simulink model "IPC4M"  (R2015a)
settings: Solver=ode3  SolverMode=SingleTasking  StartTime=0.0  StopTime=10.0  FixedStep=1e-2  RelTol=1e-7
values from neighbouring files (symbols this model uses):
  d1 = 70    [IPC4Minit.m]
  d2 = 70    [IPC4Minit.m]
  d3 = 70    [IPC4Minit.m]
  d4 = 70    [IPC4Minit.m]
  delta1 = 9    [IPC4Minit.m]
  delta2 = 9    [IPC4Minit.m]
  delta3 = 9    [IPC4Minit.m]
  delta4 = 9    [IPC4Minit.m]
  g = [0;0;-9.81]    [IPC4Minit.m]
  j0 = 10    [IPC4Minit.m]
  j1 = 10    [IPC4Minit.m]
  j1d = 1.00*j1    (= 10)    [IPC4Minit.m]
  j2 = 10    [IPC4Minit.m]
  j2d = 1.00*j2    (= 10)    [IPC4Minit.m]
  j3 = 10    [IPC4Minit.m]
  j3d = 1.00*j3    (= 10)    [IPC4Minit.m]
  j4 = 10    [IPC4Minit.m]
  j4d = 1.00*j4    (= 10)    [IPC4Minit.m]
  k1 = 2000    [IPC4Minit.m]
  k2 = 2000    [IPC4Minit.m]
  k3 = 2000    [IPC4Minit.m]
  k4 = 2000    [IPC4Minit.m]
  kappa1 = 10    [IPC4Minit.m]
  kappa2 = 10    [IPC4Minit.m]
  kappa3 = 10    [IPC4Minit.m]
  kappa4 = 10    [IPC4Minit.m]
  Kc = 150    [IPC4Minit.m]
  l = [1 1 1 1]    [IPC4Minit.m]
  m0 = 10    [IPC4Minit.m]
  m1 = 10    [IPC4Minit.m]
  m1d = 0.00*m1    (= 0)    [IPC4Minit.m]
  m2 = 10    [IPC4Minit.m]
  m2d = 0.00*m2    (= 0)    [IPC4Minit.m]
  m3 = 10    [IPC4Minit.m]
  m3d = 0.00*m3    (= 0)    [IPC4Minit.m]
  m4 = 10    [IPC4Minit.m]
  m4d = 0.00*m4    (= 0)    [IPC4Minit.m]
libraries: aerolibutil x11, dspinverses x3
(part 1 of 3)
settings Model: CovSFcnEnable=off  Creator=Martin  LastModifiedBy=mangerer
settings SolverCC: ZeroCrossAlgorithm=Adaptive
settings DataIOCC: LimitDataPoints=off
settings OptimizationCC: BlockReduction=off  BooleanDataType=off
settings DebuggingCC: SaveWithParameterizedLinksMsg=none  UnderspecifiedInitializationDetection=Classic  MergeDetectMultiDrivingBlocksExec=none  SignalResolutionControl=TryResolveAllWithWarning
settings HardwareCC: TargetUnknown=on

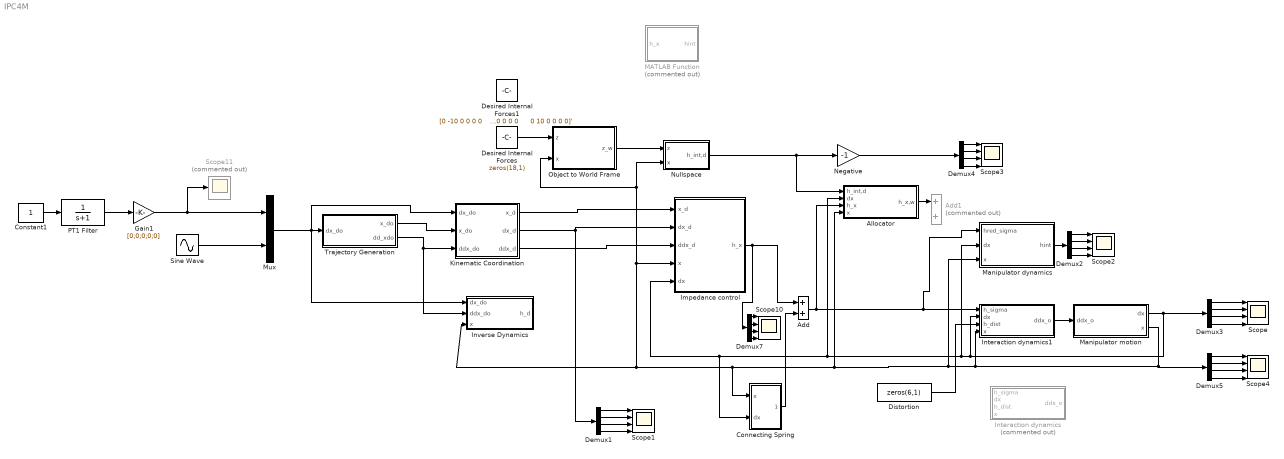
== system IPC4M ==
  Add : Sum
  Add1 : Sum  Commented=on
  Allocator : Subsystem
  Connecting Spring : Subsystem
  Constant1 : Constant
  Demux{1..5,7} (6 alike) : Demux
  Desired Internal Forces : Constant  Value=zeros(18,1)
  Desired Internal Forces1 : Constant  Value="[0 -10 0 0 0 0    10 0 0 0 0 0      0 10 0 0 0 0]'"
  Distortion : Constant  Value=zeros(6,1)
  Gain1 : Gain  Gain=[0;0;0;0;0]
  Impedance control : Subsystem
  Interaction dynamics : Subsystem  Commented=on
  Interaction dynamics1 : Subsystem
  Inverse Dynamics : Subsystem
  Kinematic Coordination : Subsystem
  MATLAB Function : MATLAB Function  Commented=on  TreatAsAtomicUnit=on
  Manipulator dynamics : Subsystem
  Manipulator motion : Subsystem
  Mux : Mux  Inputs=2
  Negative : Gain  Gain=-1
  Nullspace : Subsystem
  Object to World Frame : MATLAB Function  TreatAsAtomicUnit=on
  PT1 Filter : TransferFcn  Denominator=[1 1]
  Scope{,1..4,10} (6 alike) : Scope  NumInputPorts=4
      Scope settings: ShowLegends=on  YMin=-0.25~-0.25~-0.25~-0.25  YMax=2~2~2~2
      Scope1 settings: ShowLegends=on  YMin=-1.5~-1.5~-1.5~-1.5  YMax=6~5.5~6~5.5
      Scope10 settings: ShowLegends=on  YMin=-75~-75~-75~-75  YMax=75~75~75~75  SaveName=ScopeData18
      Scope2 settings: ShowLegends=on  YMin=-150~-150~-150~-150  YMax=150~150~150~150  SaveName=ScopeData2
      Scope3 settings: ShowLegends=on  YMin=-5~-5~-5~-5  YMax=5~5~5~5  SaveName=ScopeData8
      Scope4 settings: ShowLegends=on  YMin=-5~-5~-5~-5  YMax=5~5~5~5  SaveName=ScopeData10
  Scope11 : Scope  Commented=on
      settings: YMin=0.9984  YMax=1  SaveName=ScopeData26
  Sine Wave : Sin  Frequency=1*pi  SampleTime=0
  Trajectory Generation : Subsystem
  wires:
  Manipulator dynamics/1(hint) -> Demux2/1
  Demux2/1 -> Scope2/1
  Demux2/2 -> Scope2/2
  Demux2/4 -> Scope2/4
  Demux3/1 -> Scope/1
  Demux3/2 -> Scope/2
  Demux3/3 -> Scope/3
  Demux3/4 -> Scope/4
  Demux5/1 -> Scope4/1
  Demux5/2 -> Scope4/2
  Demux5/3 -> Scope4/3
  Demux5/4 -> Scope4/4
  Object to World Frame/1(z_w) -> Nullspace/1(z)
  Nullspace/1(h_int,d) -> Negative/1, Allocator/1(h_int,d)
  Demux7/1 -> Scope10/1
  Demux7/2 -> Scope10/2
  Demux7/3 -> Scope10/3
  Demux7/4 -> Scope10/4
  PT1 Filter/1 -> Gain1/1
  Gain1/1 -> Mux/1, Scope11/1
  Impedance control/1(h_x) -> Demux7/1, Add/1
  Manipulator motion/1(dx) -> Demux3/1, Connecting Spring/2(dx), Impedance control/5(dx), Allocator/2(dx), Manipulator dynamics/2(dx), Interaction dynamics1/2(dx)
  Trajectory Generation/2(dd_xdo) -> Inverse Dynamics/2(ddx_do), Kinematic Coordination/3(ddx_do)
  Trajectory Generation/1(x_do) -> Kinematic Coordination/2(x_do)
  Mux/1 -> Inverse Dynamics/1(dx_do), Kinematic Coordination/1(dx_do), Trajectory Generation/1(dx_do)
  Kinematic Coordination/1(x_d) -> Impedance control/1(x_d)
  Kinematic Coordination/3(ddx_d) -> Impedance control/3(ddx_d)
  Manipulator motion/2(x) -> Demux5/1, Connecting Spring/1(x), Inverse Dynamics/3(x), Object to World Frame/2(x), Nullspace/2(x), Impedance control/4(x), Allocator/4(x), Manipulator dynamics/3(x), Interaction dynamics1/4(x)
  Constant1/1 -> PT1 Filter/1
  Demux1/1 -> Scope1/1
  Demux1/2 -> Scope1/2
  Demux1/3 -> Scope1/3
  Demux1/4 -> Scope1/4
  Kinematic Coordination/2(dx_d) -> Impedance control/2(dx_d), Demux1/1
  Negative/1 -> Demux4/1
  Demux4/1 -> Scope3/1
  Demux4/2 -> Scope3/2
  Demux4/4 -> Scope3/4
  Sine Wave/1 -> Mux/2
  Demux2/3 -> Scope2/3
  Demux4/3 -> Scope3/3
  Desired Internal Forces/1 -> Object to World Frame/1(z)
  Add/1 -> Allocator/3(h_x), Manipulator dynamics/1(hred_sigma), Interaction dynamics1/1(h_sigma)
  Interaction dynamics1/1(ddx_o) -> Manipulator motion/1(ddx_o)
  Distortion/1 -> Interaction dynamics1/3(h_dist)
  Connecting Spring/1(h_con) -> Add/2
  Allocator/1(h_x,w) -> Add1/1

== system IPC4M/Allocator ==
  h_int,d : Inport
  dx : Inport  Port=2
  h_x : Inport  Port=3
  x : Inport  Port=4
  Add : Sum  Inputs=-+
  Add1 : Sum
  Divide : Product  Inputs=*/*  Multiplication=Matrix(*)
  Divide1 : Product  Inputs=*/*  Multiplication=Matrix(*)
  Divide2 : Product  Inputs=*/*  Multiplication=Matrix(*)
  Inertia : Constant  Value=blkdiag(m1d*eye(3), j1d*eye(3), m2d*eye(3), j2d*eye(3), m3d*eye(3), j3d*eye(3), m4d*eye(3), j4d*eye(3))
  MATLAB Function : MATLAB Function  TreatAsAtomicUnit=on
  MATLAB Function1 : MATLAB Function  TreatAsAtomicUnit=on
  Math Function : Math  Operator=transpose  SaturateOnIntegerOverflow=on
  h_x,w : Outport
  wires:
  dx/1 -> MATLAB Function1/1(dx)
  Divide/1 -> h_x,w/1
  Math Function/1 -> Divide1/3, Divide/1
  MATLAB Function/1(Ared) -> Math Function/1, Divide2/1, Divide1/1
  Divide1/1 -> Divide/2
  Inertia/1 -> Divide1/2, Divide2/2
  MATLAB Function1/1(bred) -> Add/2
  Add/1 -> Divide/3
  Divide2/1 -> Add/1
  Add1/1 -> Divide2/3
  h_int,d/1 -> Add1/1
  h_x/1 -> Add1/2
  x/1 -> MATLAB Function1/2(x), MATLAB Function/1(x)

== system IPC4M/Connecting Spring ==
  x : Inport
  dx : Inport  Port=2
  Add : Sum  Inputs=-+
  ConnectingDamping : MATLAB Function  TreatAsAtomicUnit=on
  ConnectingStiffness : MATLAB Function  TreatAsAtomicUnit=on
  Demux1 : Demux
  Demux6 : Demux
  Scope1 : Scope  NumInputPorts=4
      settings: ShowLegends=on  YMin=-10~-50~-80~-80  YMax=80~80~10~50  SaveName=ScopeData12
  Scope5 : Scope  NumInputPorts=4
      settings: ShowLegends=on  YMin=-10~-50~-80~-80  YMax=80~80~10~50  SaveName=ScopeData11
  h_con : Outport
  wires:
  Demux6/1 -> Scope5/1
  Demux6/2 -> Scope5/2
  Demux6/3 -> Scope5/3
  Demux6/4 -> Scope5/4
  ConnectingStiffness/1(h_con) -> Add/2, Demux6/1
  Demux1/1 -> Scope1/1
  Demux1/2 -> Scope1/2
  Demux1/3 -> Scope1/3
  Demux1/4 -> Scope1/4
  ConnectingDamping/1(h_con) -> Add/1, Demux1/1
  x/1 -> ConnectingStiffness/1(x)
  dx/1 -> ConnectingDamping/1(dx)
  Add/1 -> h_con/1

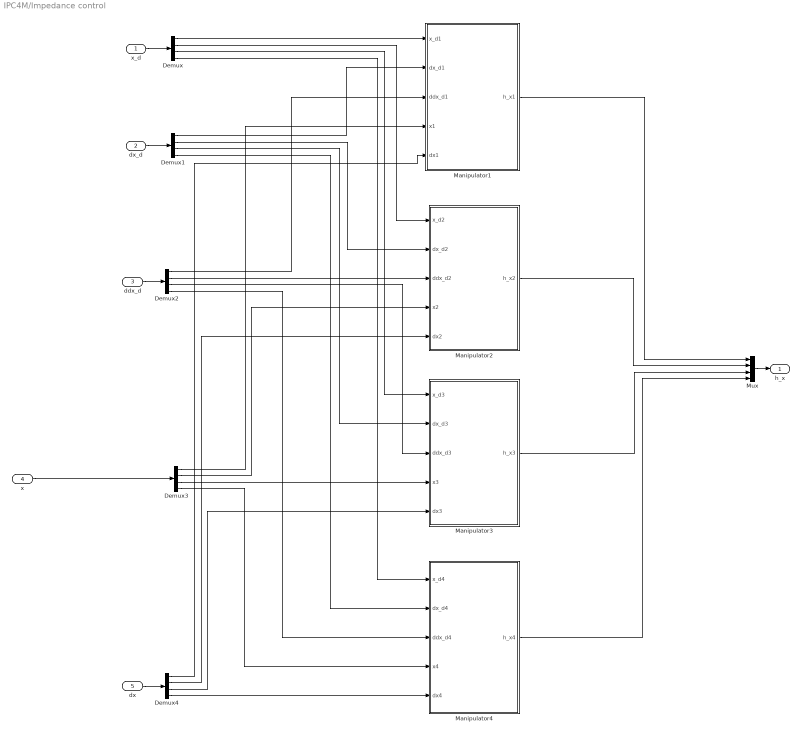
== system IPC4M/Impedance control ==
  x_d : Inport
  dx_d : Inport  Port=2
  ddx_d : Inport  Port=3
  x : Inport  Port=4
  dx : Inport  Port=5
  Demux{,1..4} (5 alike) : Demux
  Manipulator1 : Subsystem
  Manipulator2 : Subsystem
  Manipulator3 : Subsystem
  Manipulator4 : Subsystem
  Mux : Mux
  h_x : Outport
  wires:
  x/1 -> Demux3/1
  ddx_d/1 -> Demux2/1
  dx_d/1 -> Demux1/1
  x_d/1 -> Demux/1
  Demux/1 -> Manipulator1/1(x_d1)
  Demux/2 -> Manipulator2/1(x_d2)
  Demux/3 -> Manipulator3/1(x_d3)
  Demux/4 -> Manipulator4/1(x_d4)
  Demux1/1 -> Manipulator1/2(dx_d1)
  Demux1/2 -> Manipulator2/2(dx_d2)
  Demux1/3 -> Manipulator3/2(dx_d3)
  Demux1/4 -> Manipulator4/2(dx_d4)
  Demux2/1 -> Manipulator1/3(ddx_d1)
  Demux2/2 -> Manipulator2/3(ddx_d2)
  Demux2/3 -> Manipulator3/3(ddx_d3)
  Demux2/4 -> Manipulator4/3(ddx_d4)
  Demux3/1 -> Manipulator1/4(x1)
  Demux3/2 -> Manipulator2/4(x2)
  Demux3/3 -> Manipulator3/4(x3)
  Demux3/4 -> Manipulator4/4(x4)
  Demux4/4 -> Manipulator4/5(dx4)
  Demux4/3 -> Manipulator3/5(dx3)
  Demux4/2 -> Manipulator2/5(dx2)
  Demux4/1 -> Manipulator1/5(dx1)
  Mux/1 -> h_x/1
  Manipulator1/1(h_x1) -> Mux/1
  Manipulator2/1(h_x2) -> Mux/2
  Manipulator3/1(h_x3) -> Mux/3
  Manipulator4/1(h_x4) -> Mux/4
  dx/1 -> Demux4/1

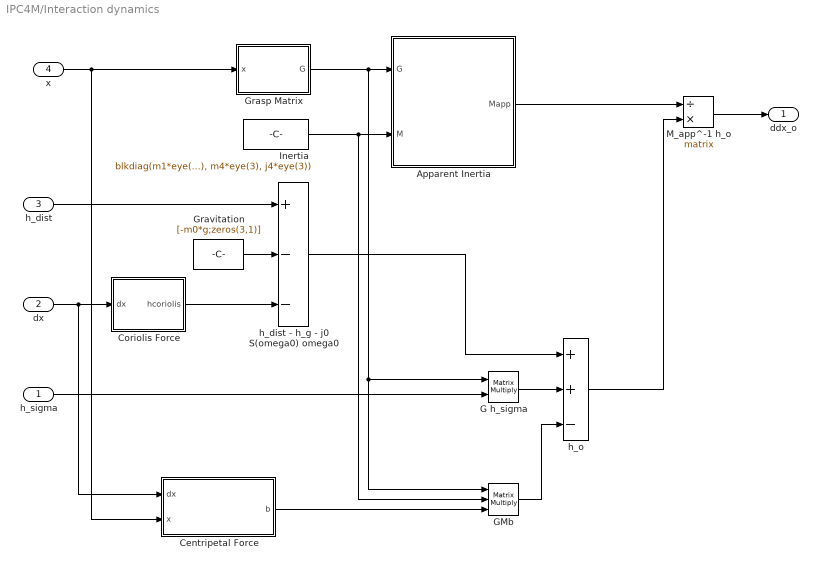
== system IPC4M/Interaction dynamics ==
  h_sigma : Inport
  dx : Inport  Port=2
  h_dist : Inport  Port=3
  x : Inport  Port=4
  Apparent Inertia : MATLAB Function  TreatAsAtomicUnit=on
  Centripetal Force : MATLAB Function  TreatAsAtomicUnit=on
  Coriolis Force : MATLAB Function  TreatAsAtomicUnit=on
  G h_sigma : Product  Multiplication=Matrix(*)
  GMb : Product  Inputs=***  Multiplication=Matrix(*)
  Grasp Matrix : MATLAB Function  TreatAsAtomicUnit=on
  Gravitation : Constant  Value=[-m0*g;zeros(3,1)]
  Inertia : Constant  Value=blkdiag(m1*eye(3), j1*eye(3), m2*eye(3), j2*eye(3), m3*eye(3), j3*eye(3), m4*eye(3), j4*eye(3))
  M_app^-1 h_o : Product  Inputs=/*  Multiplication=Matrix(*)
  "h_dist - h_g - j0 S(omega0) omega0 " : Sum  Inputs=+--
  h_o : Sum  Inputs=++-
  ddx_o : Outport
  wires:
  Grasp Matrix/1(G) -> G h_sigma/1, GMb/1, Apparent Inertia/1(G)
  Inertia/1 -> GMb/2, Apparent Inertia/2(M)
  Apparent Inertia/1(Mapp) -> M_app^-1 h_o/1
  h_o/1 -> M_app^-1 h_o/2
  G h_sigma/1 -> h_o/2
  h_sigma/1 -> G h_sigma/2
  "h_dist - h_g - j0 S(omega0) omega0 "/1 -> h_o/1
  h_dist/1 -> "h_dist - h_g - j0 S(omega0) omega0 "/1
  Gravitation/1 -> "h_dist - h_g - j0 S(omega0) omega0 "/2
  dx/1 -> Centripetal Force/1(dx), Coriolis Force/1(dx)
  Coriolis Force/1(hcoriolis) -> "h_dist - h_g - j0 S(omega0) omega0 "/3
  GMb/1 -> h_o/3
  Centripetal Force/1(b) -> GMb/3
  M_app^-1 h_o/1 -> ddx_o/1
  x/1 -> Centripetal Force/2(x), Grasp Matrix/1(x)

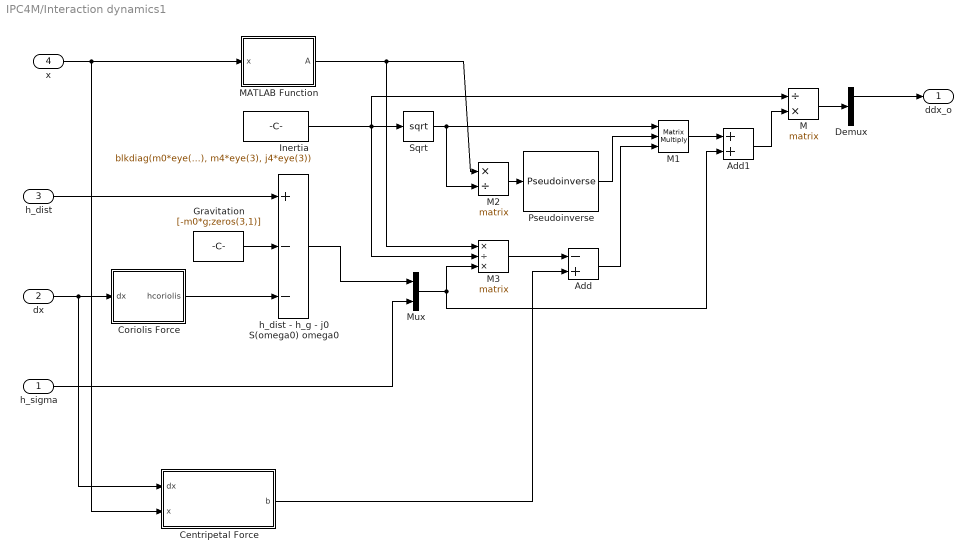
== system IPC4M/Interaction dynamics1 ==
  h_sigma : Inport
  dx : Inport  Port=2
  h_dist : Inport  Port=3
  x : Inport  Port=4
  Add : Sum  Inputs=-+
  Add1 : Sum
  Centripetal Force : MATLAB Function  TreatAsAtomicUnit=on
  Coriolis Force : MATLAB Function  TreatAsAtomicUnit=on
  Demux : Demux  Outputs=5
  Gravitation : Constant  Value=[-m0*g;zeros(3,1)]
  Inertia : Constant  Value=blkdiag(m0*eye(3),j0*eye(3),m1*eye(3), j1*eye(3), m2*eye(3), j2*eye(3), m3*eye(3), j3*eye(3), m4*eye(3), j4*eye(3))
  M : Product  Inputs=/*  Multiplication=Matrix(*)
  M1 : Product  Inputs=***  Multiplication=Matrix(*)
  M2 : Product  Inputs=*/  Multiplication=Matrix(*)
  M3 : Product  Inputs=*/*  Multiplication=Matrix(*)
  MATLAB Function : MATLAB Function  TreatAsAtomicUnit=on
  Mux : Mux  Inputs=2
  Pseudoinverse : dspinverses/Pseudoinverse  wanterr=off
  Sqrt : Sqrt  SaturateOnIntegerOverflow=on
  "h_dist - h_g - j0 S(omega0) omega0 " : Sum  Inputs=+--
  ddx_o : Outport
  wires:
  h_dist/1 -> "h_dist - h_g - j0 S(omega0) omega0 "/1
  Gravitation/1 -> "h_dist - h_g - j0 S(omega0) omega0 "/2
  dx/1 -> Centripetal Force/1(dx), Coriolis Force/1(dx)
  Coriolis Force/1(hcoriolis) -> "h_dist - h_g - j0 S(omega0) omega0 "/3
  x/1 -> MATLAB Function/1(x), Centripetal Force/2(x)
  Inertia/1 -> M/1, M3/2, Sqrt/1
  Sqrt/1 -> M2/2, M1/1
  MATLAB Function/1(A) -> M3/1, M2/1
  M2/1 -> Pseudoinverse/1
  Pseudoinverse/1 -> M1/2
  Add/1 -> M1/3
  Centripetal Force/1(b) -> Add/2
  M3/1 -> Add/1
  Mux/1 -> Add1/2, M3/3
  "h_dist - h_g - j0 S(omega0) omega0 "/1 -> Mux/1
  h_sigma/1 -> Mux/2
  M/1 -> Demux/1
  Demux/1 -> ddx_o/1
  M1/1 -> Add1/1
  Add1/1 -> M/2

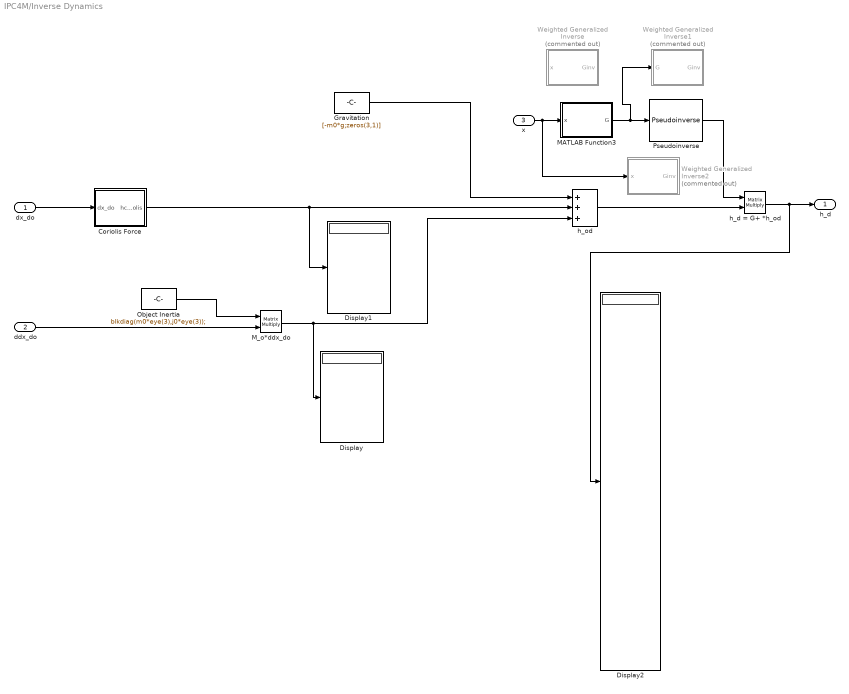
== system IPC4M/Inverse Dynamics ==
  dx_do : Inport
  ddx_do : Inport  Port=2
  x : Inport  Port=3
  Coriolis Force : MATLAB Function  TreatAsAtomicUnit=on
  Display : Display
  Display1 : Display
  Display2 : Display
  Gravitation : Constant  Value=[-m0*g;zeros(3,1)]
  MATLAB Function3 : MATLAB Function  TreatAsAtomicUnit=on
  M_o*ddx_do : Product  Multiplication=Matrix(*)
  Object Inertia : Constant  Value=blkdiag(m0*eye(3),j0*eye(3));
  Pseudoinverse : dspinverses/Pseudoinverse  wanterr=off
  Weighted Generalized Inverse : MATLAB Function  Commented=on  TreatAsAtomicUnit=on
  Weighted Generalized Inverse1 : MATLAB Function  Commented=on  TreatAsAtomicUnit=on
  Weighted Generalized Inverse2 : MATLAB Function  Commented=on  TreatAsAtomicUnit=on
  h_d = G+ *h_od : Product  Multiplication=Matrix(*)
  h_od : Sum  Inputs=+++
  h_d : Outport
  wires:
  ddx_do/1 -> M_o*ddx_do/2
  Object Inertia/1 -> M_o*ddx_do/1
  dx_do/1 -> Coriolis Force/1(dx_do)
  Gravitation/1 -> h_od/1
  MATLAB Function3/1(G) -> Weighted Generalized Inverse1/1(G), Pseudoinverse/1
  h_d = G+ *h_od/1 -> Display2/1, h_d/1
  x/1 -> Weighted Generalized Inverse2/1(x), MATLAB Function3/1(x)
  M_o*ddx_do/1 -> Display/1, h_od/3
  h_od/1 -> h_d = G+ *h_od/2
  Coriolis Force/1(hcoriolis) -> Display1/1, h_od/2
  Pseudoinverse/1 -> h_d = G+ *h_od/1

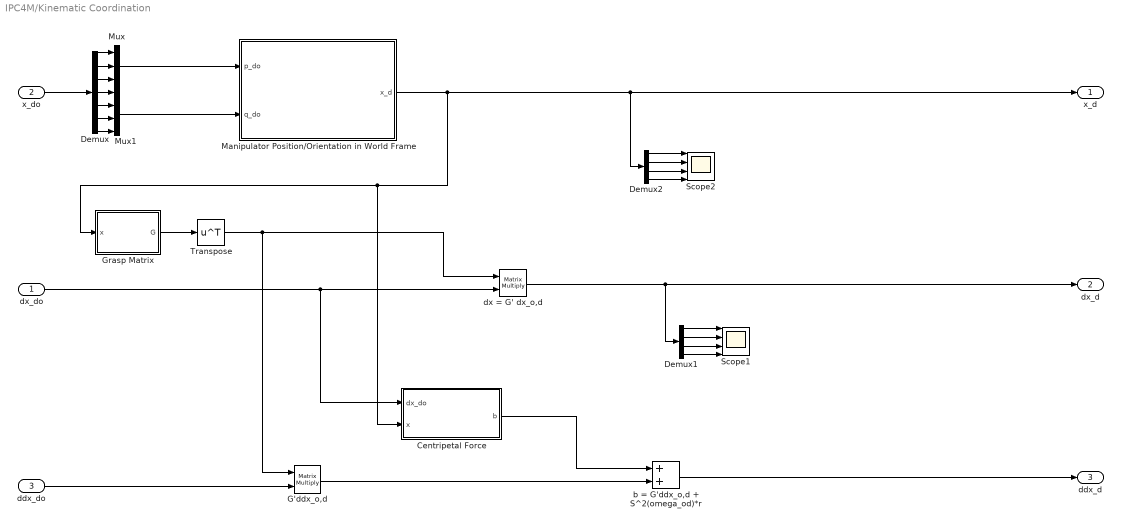
== system IPC4M/Kinematic Coordination ==
  dx_do : Inport
  x_do : Inport  Port=2
  ddx_do : Inport  Port=3
  Centripetal Force : MATLAB Function  TreatAsAtomicUnit=on
  Demux : Demux  Outputs=7
  Demux1 : Demux
  Demux2 : Demux
  G'ddx_o,d : Product  Multiplication=Matrix(*)
  Grasp Matrix : MATLAB Function  TreatAsAtomicUnit=on
  Manipulator Position/Orientation in World Frame : MATLAB Function  TreatAsAtomicUnit=on
  Mux : Mux  Inputs=3
  Mux1 : Mux
  Scope1 : Scope  NumInputPorts=4
      settings: ShowLegends=on  YMin=-1.5~-1.5~-1.5~-1.5  YMax=6~5.5~6~5.5  SaveName=ScopeData3
  Scope2 : Scope  NumInputPorts=4
      settings: ShowLegends=on  YMin=-1.5~-1.5~-1.5~-1.5  YMax=6~5.5~6~5.5  SaveName=ScopeData4
  Transpose : Math  Operator=transpose  SaturateOnIntegerOverflow=on
  b = G'ddx_o,d + S^2(omega_od)*r : Sum
  dx = G' dx_o,d : Product  Multiplication=Matrix(*)
  x_d : Outport
  dx_d : Outport  Port=2
  ddx_d : Outport  Port=3
  wires:
  Grasp Matrix/1(G) -> Transpose/1
  Transpose/1 -> G'ddx_o,d/1, dx = G' dx_o,d/1
  dx = G' dx_o,d/1 -> Demux1/1, dx_d/1
  x_do/1 -> Demux/1
  Demux/1 -> Mux/1
  Demux/2 -> Mux/2
  Demux/3 -> Mux/3
  Demux/5 -> Mux1/2
  Demux/6 -> Mux1/3
  Demux/7 -> Mux1/4
  Demux/4 -> Mux1/1
  Mux1/1 -> Manipulator Position/Orientation in World Frame/2(q_do)
  Mux/1 -> Manipulator Position/Orientation in World Frame/1(p_do)
  Centripetal Force/1(b) -> b = G'ddx_o,d + S^2(omega_od)*r/1
  ddx_do/1 -> G'ddx_o,d/2
  G'ddx_o,d/1 -> b = G'ddx_o,d + S^2(omega_od)*r/2
  b = G'ddx_o,d + S^2(omega_od)*r/1 -> ddx_d/1
  dx_do/1 -> Centripetal Force/1(dx_do), dx = G' dx_o,d/2
  Demux1/1 -> Scope1/1
  Demux1/2 -> Scope1/2
  Demux1/3 -> Scope1/3
  Demux1/4 -> Scope1/4
  Manipulator Position/Orientation in World Frame/1(x_d) -> Centripetal Force/2(x), Grasp Matrix/1(x), Demux2/1, x_d/1
  Demux2/1 -> Scope2/1
  Demux2/2 -> Scope2/2
  Demux2/3 -> Scope2/3
  Demux2/4 -> Scope2/4

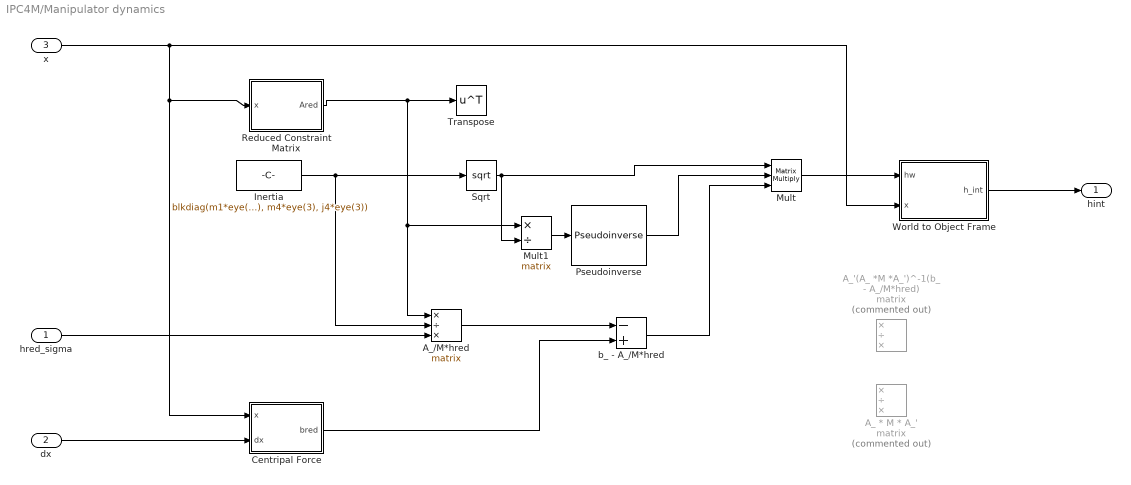
== system IPC4M/Manipulator dynamics ==
  hred_sigma : Inport
  dx : Inport  Port=2
  x : Inport  Port=3
  A_ * M * A_' : Product  Commented=on  Inputs=*/*  Multiplication=Matrix(*)
  A_'(A_ *M *A_')^-1(b_ - A_/M*hred) : Product  Commented=on  Inputs=*/*  Multiplication=Matrix(*)
  A_/M*hred : Product  Inputs=*/*  Multiplication=Matrix(*)
  Centripal Force : MATLAB Function  TreatAsAtomicUnit=on
  Inertia : Constant  Value=blkdiag(m1*eye(3), j1*eye(3), m2*eye(3), j2*eye(3), m3*eye(3), j3*eye(3), m4*eye(3), j4*eye(3))
  Mult : Product  Inputs=***  Multiplication=Matrix(*)
  Mult1 : Product  Inputs=*/  Multiplication=Matrix(*)
  Pseudoinverse : dspinverses/Pseudoinverse  wanterr=off
  Reduced Constraint Matrix : MATLAB Function  TreatAsAtomicUnit=on
  Sqrt : Sqrt  SaturateOnIntegerOverflow=on
  Transpose : Math  Operator=transpose  SaturateOnIntegerOverflow=on
  World to Object Frame : MATLAB Function  TreatAsAtomicUnit=on
  b_ - A_/M*hred : Sum  Inputs=-+
  hint : Outport
  wires:
  Reduced Constraint Matrix/1(Ared) -> Transpose/1, A_/M*hred/1, Mult1/1
  Inertia/1 -> Sqrt/1, A_/M*hred/2
  dx/1 -> Centripal Force/2(dx)
  A_/M*hred/1 -> b_ - A_/M*hred/1
  hred_sigma/1 -> A_/M*hred/3
  World to Object Frame/1(h_int) -> hint/1
  x/1 -> Centripal Force/1(x), Reduced Constraint Matrix/1(x), World to Object Frame/2(x)
  Centripal Force/1(bred) -> b_ - A_/M*hred/2
  Mult/1 -> World to Object Frame/1(hw)
  b_ - A_/M*hred/1 -> Mult/3
  Sqrt/1 -> Mult1/2, Mult/1
  Mult1/1 -> Pseudoinverse/1
  Pseudoinverse/1 -> Mult/2

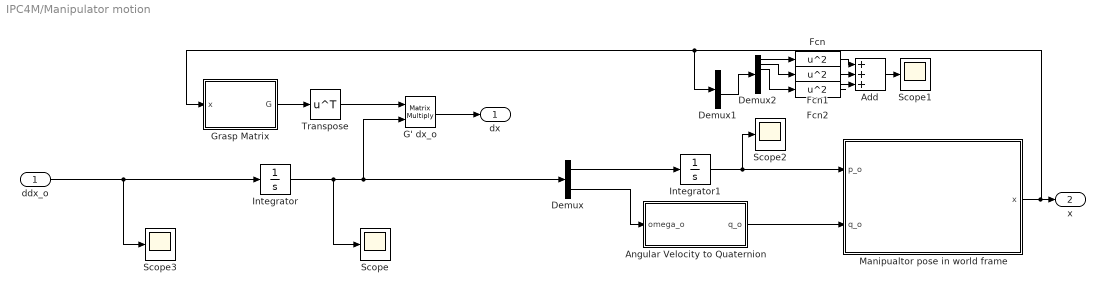
== system IPC4M/Manipulator motion ==
  ddx_o : Inport
  Add : Sum  Inputs=+++
  Angular Velocity to Quaternion : Subsystem
  Demux : Demux  Outputs=2
  Demux1 : Demux
  Demux2 : Demux  Outputs=7
  Fcn : Fcn  Expr=u^2
  Fcn1 : Fcn  Expr=u^2
  Fcn2 : Fcn  Expr=u^2
  G' dx_o : Product  Multiplication=Matrix(*)
  Grasp Matrix : MATLAB Function  TreatAsAtomicUnit=on
  Integrator : Integrator  InitialCondition=zeros(6,1)
  Integrator1 : Integrator  InitialCondition=[0 0 0]'
  Manipualtor pose in world frame : MATLAB Function  TreatAsAtomicUnit=on
  Scope{,1..3} (4 alike) : Scope
      Scope settings: SaveName=ScopeData14
      Scope1 settings: YMin=0.7  YMax=0.9  SaveName=ScopeData15
      Scope2 settings: YMin=-1  YMax=1  SaveName=ScopeData6
      Scope3 settings: SaveName=ScopeData7
  Transpose : Math  Operator=transpose  SaturateOnIntegerOverflow=on
  dx : Outport
  x : Outport  Port=2
  wires:
  ddx_o/1 -> Scope3/1, Integrator/1
  Integrator/1 -> Scope/1, G' dx_o/2, Demux/1
  Grasp Matrix/1(G) -> Transpose/1
  Transpose/1 -> G' dx_o/1
  G' dx_o/1 -> dx/1
  Demux/2 -> Angular Velocity to Quaternion/1(omega_o)
  Demux/1 -> Integrator1/1
  Integrator1/1 -> Scope2/1, Manipualtor pose in world frame/1(p_o)
  Manipualtor pose in world frame/1(x) -> Demux1/1, Grasp Matrix/1(x), x/1
  Angular Velocity to Quaternion/1(q_o) -> Manipualtor pose in world frame/2(q_o)
  Add/1 -> Scope1/1
  Fcn/1 -> Add/1
  Fcn1/1 -> Add/2
  Fcn2/1 -> Add/3
  Demux2/1 -> Fcn/1
  Demux2/2 -> Fcn1/1
  Demux2/3 -> Fcn2/1
  Demux1/3 -> Demux2/1

== system IPC4M/Nullspace ==
  z : Inport
  x : Inport  Port=2
  A_' * z : Product  Multiplication=Matrix(*)
  Reduced Constraint Matrix : MATLAB Function  TreatAsAtomicUnit=on
  Transpose : Math  Operator=transpose  SaturateOnIntegerOverflow=on
  h_int,d : Outport
  wires:
  Reduced Constraint Matrix/1(Ared) -> Transpose/1
  Transpose/1 -> A_' * z/1
  z/1 -> A_' * z/2
  A_' * z/1 -> h_int,d/1
  x/1 -> Reduced Constraint Matrix/1(x)

== system IPC4M/Trajectory Generation ==
  dx_do : Inport
  Angular Velocity to Quaternion Orientation : Subsystem
  Demux : Demux  Outputs=2
  Derivative : Derivative
  Integrator : Integrator  InitialCondition=zeros(3,1)
  Mux : Mux  Inputs=2
  Quaternion Normalize : aerolibutil/Quaternion Normalize
  x_do : Outport
  dd_xdo : Outport  Port=2
  wires:
  dx_do/1 -> Derivative/1, Demux/1
  Demux/2 -> Angular Velocity to Quaternion Orientation/1(omega_do)
  Demux/1 -> Integrator/1
  Angular Velocity to Quaternion Orientation/1(q_do) -> Quaternion Normalize/1
  Integrator/1 -> Mux/1
  Mux/1 -> x_do/1
  Derivative/1 -> dd_xdo/1
  Quaternion Normalize/1 -> Mux/2

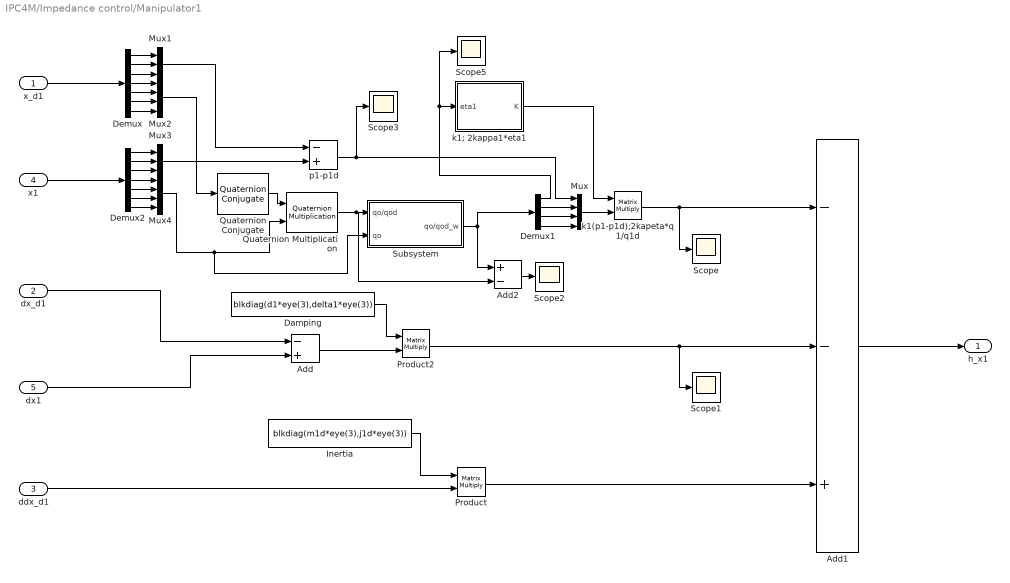
== system IPC4M/Impedance control/Manipulator1 ==
  x_d1 : Inport
  dx_d1 : Inport  Port=2
  ddx_d1 : Inport  Port=3
  x1 : Inport  Port=4
  dx1 : Inport  Port=5
  Add : Sum  Inputs=-+
  Add1 : Sum  Inputs=--+
  Add2 : Sum  Inputs=+-
  Damping : Constant  Value=blkdiag(d1*eye(3),delta1*eye(3))
  Demux : Demux  Outputs=7
  Demux1 : Demux
  Demux2 : Demux  Outputs=7
  Inertia : Constant  Value=blkdiag(m1d*eye(3),j1d*eye(3))
  Mux : Mux
  Mux1 : Mux  Inputs=3
  Mux2 : Mux
  Mux3 : Mux  Inputs=3
  Mux4 : Mux
  Product : Product  Multiplication=Matrix(*)
  Product2 : Product  Multiplication=Matrix(*)
  Quaternion Conjugate : aerolibutil/Quaternion Conjugate
  Quaternion Multiplication : aerolibutil/Quaternion Multiplication
  Scope{,1..3,5} (5 alike) : Scope
      Scope settings: TimeRange=200  YMin=-50  YMax=125  SaveName=ScopeData13
      Scope1 settings: TimeRange=200  YMin=-50  YMax=125  SaveName=ScopeData19
      Scope2 settings: SaveName=ScopeData5
      Scope3 settings: ShowLegends=on  TimeRange=200  YMin=-50  YMax=125  SaveName=ScopeData21
      Scope5 settings: ShowLegends=on  TimeRange=200  YMin=-50  YMax=125  SaveName=ScopeData24
  Subsystem : Subsystem
  k1(p1-p1d);2kapeta*q1/q1d : Product  Multiplication=Matrix(*)
  k1; 2kappa1*eta1 : MATLAB Function  TreatAsAtomicUnit=on
  p1-p1d : Sum  Inputs=-+
  h_x1 : Outport
  wires:
  Add/1 -> Product2/2
  Damping/1 -> Product2/1
  dx_d1/1 -> Add/1
  dx1/1 -> Add/2
  k1; 2kappa1*eta1/1(K) -> k1(p1-p1d);2kapeta*q1/q1d/1
  Demux1/1 -> Scope5/1, k1; 2kappa1*eta1/1(eta1)
  p1-p1d/1 -> Scope3/1, Mux/1
  Demux1/2 -> Mux/2
  Demux1/3 -> Mux/3
  Demux1/4 -> Mux/4
  x1/1 -> Demux2/1
  x_d1/1 -> Demux/1
  Demux/2 -> Mux1/2
  Demux/1 -> Mux1/1
  Demux/3 -> Mux1/3
  Demux/4 -> Mux2/1
  Demux/5 -> Mux2/2
  Demux/6 -> Mux2/3
  Demux/7 -> Mux2/4
  Demux2/2 -> Mux3/2
  Demux2/1 -> Mux3/1
  Demux2/3 -> Mux3/3
  Demux2/4 -> Mux4/1
  Demux2/5 -> Mux4/2
  Demux2/6 -> Mux4/3
  Demux2/7 -> Mux4/4
  Mux1/1 -> p1-p1d/1
  Mux3/1 -> p1-p1d/2
  Inertia/1 -> Product/1
  Add1/1 -> h_x1/1
  k1(p1-p1d);2kapeta*q1/q1d/1 -> Scope/1, Add1/1
  Product2/1 -> Scope1/1, Add1/2
  Product/1 -> Add1/3
  ddx_d1/1 -> Product/2
  Mux4/1 -> Quaternion Multiplication/2, Subsystem/2(qo)
  Mux/1 -> k1(p1-p1d);2kapeta*q1/q1d/2
  Quaternion Multiplication/1 -> Add2/2, Subsystem/1(qo/qod)
  Subsystem/1(qo/qod_w) -> Add2/1, Demux1/1
  Add2/1 -> Scope2/1
  Mux2/1 -> Quaternion Conjugate/1
  Quaternion Conjugate/1 -> Quaternion Multiplication/1

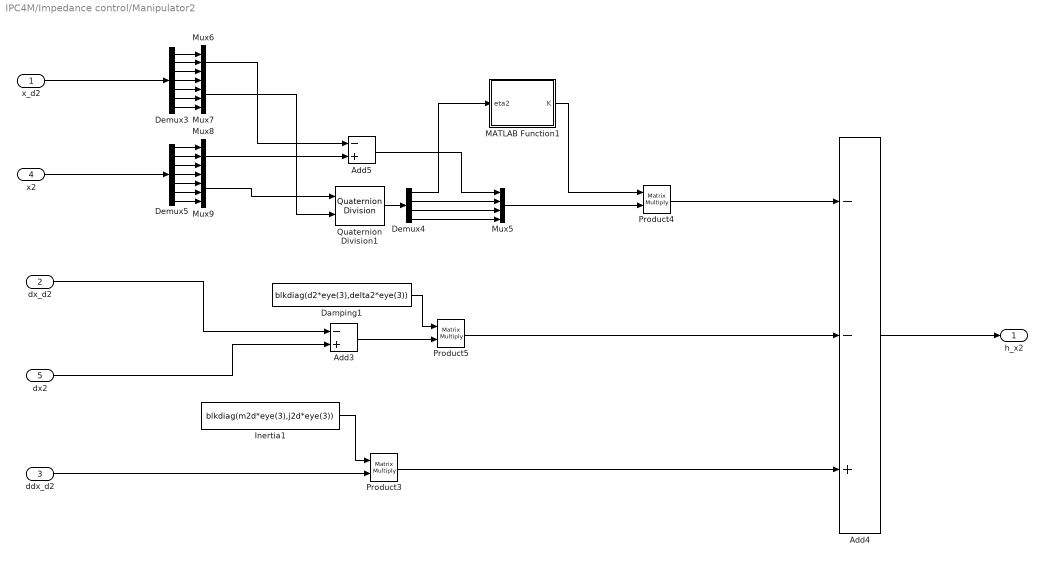
== system IPC4M/Impedance control/Manipulator2 ==
  x_d2 : Inport
  dx_d2 : Inport  Port=2
  ddx_d2 : Inport  Port=3
  x2 : Inport  Port=4
  dx2 : Inport  Port=5
  Add3 : Sum  Inputs=-+
  Add4 : Sum  Inputs=--+
  Add5 : Sum  Inputs=-+
  Damping1 : Constant  Value=blkdiag(d2*eye(3),delta2*eye(3))
  Demux3 : Demux  Outputs=7
  Demux4 : Demux
  Demux5 : Demux  Outputs=7
  Inertia1 : Constant  Value=blkdiag(m2d*eye(3),j2d*eye(3))
  MATLAB Function1 : MATLAB Function  TreatAsAtomicUnit=on
  Mux5 : Mux
  Mux6 : Mux  Inputs=3
  Mux7 : Mux
  Mux8 : Mux  Inputs=3
  Mux9 : Mux
  Product3 : Product  Multiplication=Matrix(*)
  Product4 : Product  Multiplication=Matrix(*)
  Product5 : Product  Multiplication=Matrix(*)
  Quaternion Division1 : aerolibutil/Quaternion Division
  h_x2 : Outport
  wires:
  Add3/1 -> Product5/2
  Damping1/1 -> Product5/1
  dx_d2/1 -> Add3/1
  dx2/1 -> Add3/2
  MATLAB Function1/1(K) -> Product4/1
  Demux4/1 -> MATLAB Function1/1(eta2)
  Add5/1 -> Mux5/1
  Demux4/2 -> Mux5/2
  Demux4/3 -> Mux5/3
  Demux4/4 -> Mux5/4
  x2/1 -> Demux5/1
  x_d2/1 -> Demux3/1
  Demux3/2 -> Mux6/2
  Demux3/1 -> Mux6/1
  Demux3/3 -> Mux6/3
  Demux3/4 -> Mux7/1
  Demux3/5 -> Mux7/2
  Demux3/6 -> Mux7/3
  Demux3/7 -> Mux7/4
  Demux5/2 -> Mux8/2
  Demux5/1 -> Mux8/1
  Demux5/3 -> Mux8/3
  Demux5/4 -> Mux9/1
  Demux5/5 -> Mux9/2
  Demux5/6 -> Mux9/3
  Demux5/7 -> Mux9/4
  Mux6/1 -> Add5/1
  Mux8/1 -> Add5/2
  Quaternion Division1/1 -> Demux4/1
  Mux5/1 -> Product4/2
  Inertia1/1 -> Product3/1
  Add4/1 -> h_x2/1
  Product4/1 -> Add4/1
  Product5/1 -> Add4/2
  Product3/1 -> Add4/3
  ddx_d2/1 -> Product3/2
  Mux7/1 -> Quaternion Division1/2
  Mux9/1 -> Quaternion Division1/1

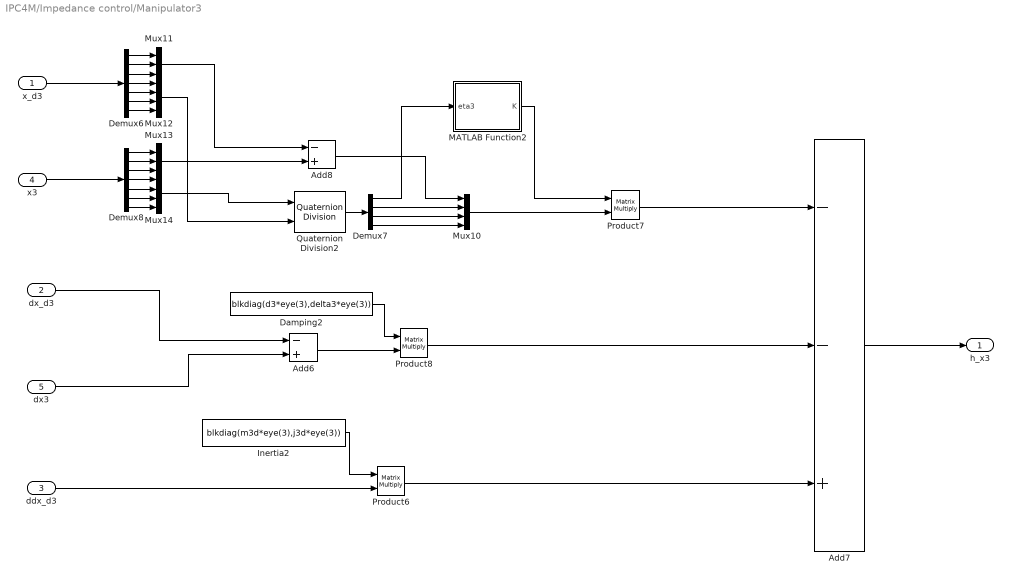
== system IPC4M/Impedance control/Manipulator3 ==
  x_d3 : Inport
  dx_d3 : Inport  Port=2
  ddx_d3 : Inport  Port=3
  x3 : Inport  Port=4
  dx3 : Inport  Port=5
  Add6 : Sum  Inputs=-+
  Add7 : Sum  Inputs=--+
  Add8 : Sum  Inputs=-+
  Damping2 : Constant  Value=blkdiag(d3*eye(3),delta3*eye(3))
  Demux6 : Demux  Outputs=7
  Demux7 : Demux
  Demux8 : Demux  Outputs=7
  Inertia2 : Constant  Value=blkdiag(m3d*eye(3),j3d*eye(3))
  MATLAB Function2 : MATLAB Function  TreatAsAtomicUnit=on
  Mux10 : Mux
  Mux11 : Mux  Inputs=3
  Mux12 : Mux
  Mux13 : Mux  Inputs=3
  Mux14 : Mux
  Product6 : Product  Multiplication=Matrix(*)
  Product7 : Product  Multiplication=Matrix(*)
  Product8 : Product  Multiplication=Matrix(*)
  Quaternion Division2 : aerolibutil/Quaternion Division
  h_x3 : Outport
  wires:
  Add6/1 -> Product8/2
  Damping2/1 -> Product8/1
  dx_d3/1 -> Add6/1
  dx3/1 -> Add6/2
  MATLAB Function2/1(K) -> Product7/1
  Demux7/1 -> MATLAB Function2/1(eta3)
  Add8/1 -> Mux10/1
  Demux7/2 -> Mux10/2
  Demux7/3 -> Mux10/3
  Demux7/4 -> Mux10/4
  x3/1 -> Demux8/1
  x_d3/1 -> Demux6/1
  Demux6/2 -> Mux11/2
  Demux6/1 -> Mux11/1
  Demux6/3 -> Mux11/3
  Demux6/4 -> Mux12/1
  Demux6/5 -> Mux12/2
  Demux6/6 -> Mux12/3
  Demux6/7 -> Mux12/4
  Demux8/2 -> Mux13/2
  Demux8/1 -> Mux13/1
  Demux8/3 -> Mux13/3
  Demux8/4 -> Mux14/1
  Demux8/5 -> Mux14/2
  Demux8/6 -> Mux14/3
  Demux8/7 -> Mux14/4
  Mux11/1 -> Add8/1
  Mux13/1 -> Add8/2
  Quaternion Division2/1 -> Demux7/1
  Mux10/1 -> Product7/2
  Inertia2/1 -> Product6/1
  Add7/1 -> h_x3/1
  Product7/1 -> Add7/1
  Product8/1 -> Add7/2
  Product6/1 -> Add7/3
  ddx_d3/1 -> Product6/2
  Mux14/1 -> Quaternion Division2/1
  Mux12/1 -> Quaternion Division2/2

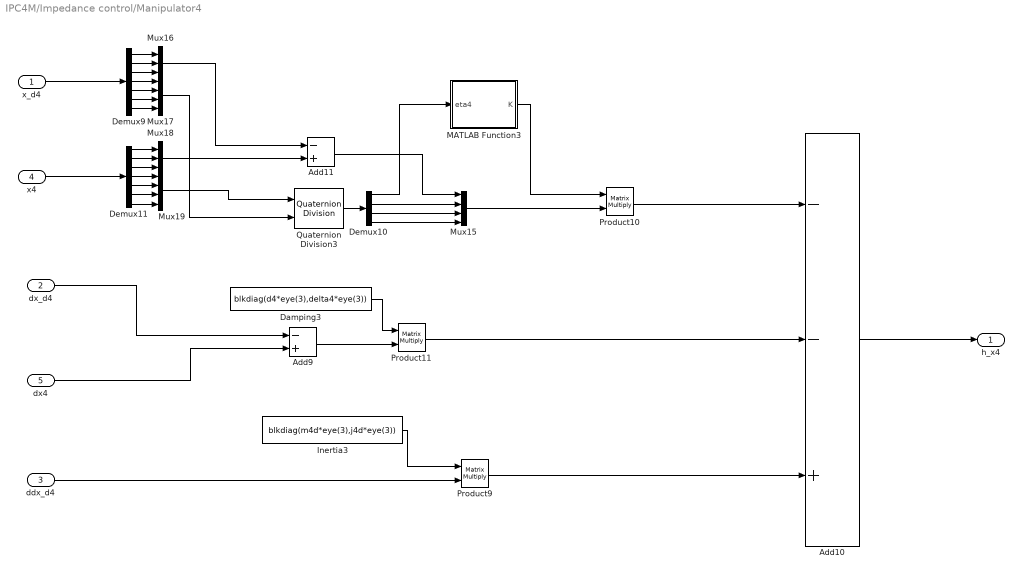
== system IPC4M/Impedance control/Manipulator4 ==
  x_d4 : Inport
  dx_d4 : Inport  Port=2
  ddx_d4 : Inport  Port=3
  x4 : Inport  Port=4
  dx4 : Inport  Port=5
  Add10 : Sum  Inputs=--+
  Add11 : Sum  Inputs=-+
  Add9 : Sum  Inputs=-+
  Damping3 : Constant  Value=blkdiag(d4*eye(3),delta4*eye(3))
  Demux10 : Demux
  Demux11 : Demux  Outputs=7
  Demux9 : Demux  Outputs=7
  Inertia3 : Constant  Value=blkdiag(m4d*eye(3),j4d*eye(3))
  MATLAB Function3 : MATLAB Function  TreatAsAtomicUnit=on
  Mux15 : Mux
  Mux16 : Mux  Inputs=3
  Mux17 : Mux
  Mux18 : Mux  Inputs=3
  Mux19 : Mux
  Product10 : Product  Multiplication=Matrix(*)
  Product11 : Product  Multiplication=Matrix(*)
  Product9 : Product  Multiplication=Matrix(*)
  Quaternion Division3 : aerolibutil/Quaternion Division
  h_x4 : Outport
  wires:
  Add9/1 -> Product11/2
  Damping3/1 -> Product11/1
  dx_d4/1 -> Add9/1
  dx4/1 -> Add9/2
  MATLAB Function3/1(K) -> Product10/1
  Demux10/1 -> MATLAB Function3/1(eta4)
  Add11/1 -> Mux15/1
  Demux10/2 -> Mux15/2
  Demux10/3 -> Mux15/3
  Demux10/4 -> Mux15/4
  x4/1 -> Demux11/1
  x_d4/1 -> Demux9/1
  Demux9/2 -> Mux16/2
  Demux9/1 -> Mux16/1
  Demux9/3 -> Mux16/3
  Demux9/4 -> Mux17/1
  Demux9/5 -> Mux17/2
  Demux9/6 -> Mux17/3
  Demux9/7 -> Mux17/4
  Demux11/2 -> Mux18/2
  Demux11/1 -> Mux18/1
  Demux11/3 -> Mux18/3
  Demux11/4 -> Mux19/1
  Demux11/5 -> Mux19/2
  Demux11/6 -> Mux19/3
  Demux11/7 -> Mux19/4
  Mux16/1 -> Add11/1
  Mux18/1 -> Add11/2
  Quaternion Division3/1 -> Demux10/1
  Mux15/1 -> Product10/2
  Inertia3/1 -> Product9/1
  Add10/1 -> h_x4/1
  Product10/1 -> Add10/1
  Product11/1 -> Add10/2
  Product9/1 -> Add10/3
  ddx_d4/1 -> Product9/2
  Mux19/1 -> Quaternion Division3/1
  Mux17/1 -> Quaternion Division3/2

== system IPC4M/Manipulator motion/Angular Velocity to Quaternion ==
  omega_o : Inport
  Constant : Constant  Value=0
  Gain : Gain  Gain=0.5
  Integrator : Integrator  InitialCondition=[1; 0; 0; 0]
  Mux : Mux  Inputs=2
  Quaternion Multiplication : aerolibutil/Quaternion Multiplication
  Scope : Scope
      settings: ShowLegends=on  SaveName=ScopeData9
  q_o : Outport
  wires:
  omega_o/1 -> Gain/1
  Gain/1 -> Mux/2
  Constant/1 -> Mux/1
  Quaternion Multiplication/1 -> Integrator/1
  Integrator/1 -> Quaternion Multiplication/2, q_o/1, Scope/1
  Mux/1 -> Quaternion Multiplication/1

== system IPC4M/Trajectory Generation/Angular Velocity to Quaternion Orientation ==
  omega_do : Inport
  Constant : Constant  Value=0
  Gain : Gain  Gain=0.5
  Integrator : Integrator  InitialCondition=[1; 0; 0; 0]
  Mux : Mux  Inputs=2
  Quaternion Multiplication : aerolibutil/Quaternion Multiplication
  Scope : Scope
      settings: ShowLegends=on  SaveName=ScopeData9
  q_do : Outport
  wires:
  omega_do/1 -> Gain/1
  Gain/1 -> Mux/2
  Constant/1 -> Mux/1
  Quaternion Multiplication/1 -> Integrator/1
  Integrator/1 -> Quaternion Multiplication/2, Scope/1, q_do/1
  Mux/1 -> Quaternion Multiplication/1

== system IPC4M/Impedance control/Manipulator1/Subsystem ==
  qo/qod : Inport
  qo : Inport  Port=2
  Quaternion Conjugate1 : aerolibutil/Quaternion Conjugate
  Quaternion Multiplication1 : aerolibutil/Quaternion Multiplication
  Quaternion Multiplication2 : aerolibutil/Quaternion Multiplication
  qo/qod_w : Outport
  wires:
  qo/1 -> Quaternion Conjugate1/1, Quaternion Multiplication1/1
  Quaternion Multiplication2/1 -> Quaternion Multiplication1/2
  qo/qod/1 -> Quaternion Multiplication2/1
  Quaternion Conjugate1/1 -> Quaternion Multiplication2/2
  Quaternion Multiplication1/1 -> qo/qod_w/1

== matlab function IPC4M/Inverse Dynamics/Coriolis Force ==
  data: dx_do input; hcoriolis output; j0 parameter; m0 parameter
function hcoriolis = CoriolisForce(dx_do,j0,m0)
hcoriolis = [m0*skew_sm(dx_do(4:6))*dx_do(1:3);
        j0*skew_sm(dx_do(4:6))*dx_do(4:6)];

== matlab function IPC4M/Inverse Dynamics/Weighted Generalized Inverse ==
  data: x input; Ginv output; r parameter
function Ginv = GraspInverse(x,r)
J = eye(3) + 0.25 * (skew_sm(quatrot(x(4:7),r(1:3)))*skew_sm(quatrot(x(4:7),r(1:3)))' + skew_sm(quatrot(x(4:7),r(4:6)))*skew_sm(quatrot(x(4:7),r(4:6)))' + skew_sm(quatrot(x(4:7),r(7:9)))*skew_sm(quatrot(x(4:7),r(7:9)))' + skew_sm(quatrot(x(4:7),r(10:12)))*skew_sm(quatrot(x(4:7),r(10:12)))');
Jinv = J^-1;
Ginv = 0.25*[eye(3) Jinv*skew_sm(quatrot(x(4:7),r(1:3)))';
             zeros(3) Jinv;
             eye(3) Jinv*skew_sm(quatrot(x(4:7),r(4:6)))';
             zeros(3) Jinv;
             eye(3) Jinv*skew_sm(quatrot(x(4:7),r(7:9)))';
             zeros(3) Jinv;
             eye(3) Jinv*skew_sm(quatrot(x(4:7),r(10:12)))';
             zeros(3) Jinv];

== matlab function IPC4M/Inverse Dynamics/Weighted Generalized Inverse1 ==
  data: G input; Ginv output
function Ginv = MATLABpinv(G)
Ginv = pinv(G);
